simulink model "SimpleMass"  (R2018a)
settings: Solver=VariableStepAuto  StartTime=0.0  StopTime=Ttot  MaxStep=0.1  RelTol=1e-3
values from neighbouring files (symbols this model uses):
  DeadTimeValve = 0.1    [SimpleMass_Script.m]
  J = 2 * H * Sn / omegan^2    (= 4458.13208026)    [SimpleMass_Script.m]
  kgov = kgov_WHz / Sn * Fn    (= 5)    [SimpleMass_Script.m]
  Kpsec = 0    [SimpleMass_Script.m]
  omegan = 2 * pi * Fn / np    (= 314.159265359)    [SimpleMass_Script.m]
  Peini = 44e6/Sn    (= 0.5)    [SimpleMass_Script.m]
  Pestep = 4.4e6/Sn    (= 0.05)    [SimpleMass_Script.m]
  Sn = 2*44e6    (= 88000000)    [SimpleMass_Script.m]
  StepTime = 10    [SimpleMass_Script.m]
  Tgt1 = 0.1    [SimpleMass_Script.m]
  Tgt2 = 0.4    [SimpleMass_Script.m]
  Tsec = 4    [SimpleMass_Script.m]
  Tsec_on_delay = 25    [SimpleMass_Script.m]
undefined symbols (not defined in the file or in its folder): RateSec
settings Model: Creator=daniemot  LastModifiedBy=daniemot

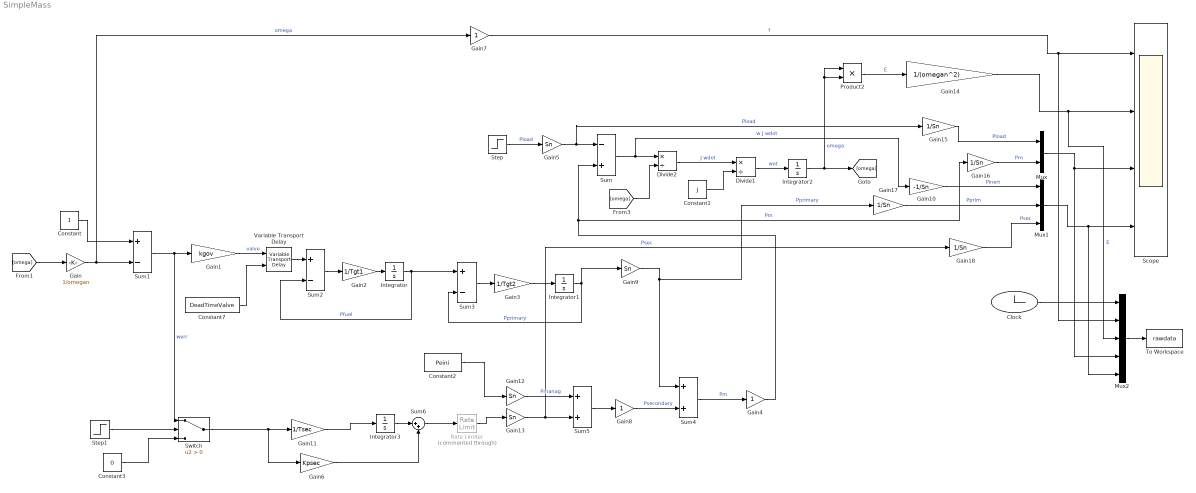
== system SimpleMass ==
  Clock : Clock
  Constant : Constant
  Constant1 : Constant  Value=J
  Constant2 : Constant  Value=Peini
  Constant3 : Constant  Value=0
  Constant7 : Constant  Value=DeadTimeValve
  Divide1 : Product  Inputs=*/
  Divide2 : Product  Inputs=*/
  Gain : Gain  Gain=1/omegan
  Gain1 : Gain  Gain=kgov
  Gain10 : Gain  Gain=-1/Sn
  Gain11 : Gain  Gain=1/Tsec
  Gain{5,9,12..13} (4 alike) : Gain  Gain=Sn
  Gain14 : Gain  Gain=1/(omegan^2)
  Gain{15..18} (4 alike) : Gain  Gain=1/Sn
  Gain2 : Gain  Gain=1/Tgt1
  Gain3 : Gain  Gain=1/Tgt2
  Gain4 : Gain
  Gain6 : Gain  Gain=Kpsec
  Gain7 : Gain
  Gain8 : Gain
  Integrator : Integrator
  Integrator1 : Integrator
  Integrator2 : Integrator  InitialCondition=omegan
  Integrator3 : Integrator
  Mux : Mux  Inputs=2
  Mux1 : Mux  Inputs=3
  Mux2 : Mux  Inputs=5
  Product2 : Product
  Rate Limiter : RateLimiter  Commented=through  RisingSlewLimit=RateSec  FallingSlewLimit=-RateSec  SampleTimeMode=inherited
  Scope : Scope  NumInputPorts=4
  Step : Step  Time=StepTime  Before=Peini  After=Peini + Pestep  SampleTime=0
  Step1 : Step  Time=Tsec_on_delay  SampleTime=0
  Sum : Sum  Inputs=-+
  Sum1 : Sum  Inputs=+-
  Sum2 : Sum  Inputs=+-
  Sum3 : Sum  Inputs=+-
  Sum4 : Sum
  Sum5 : Sum
  Sum6 : Sum  Inputs=|++
  Switch : Switch  Criteria=u2 > Threshold
  To Workspace : ToWorkspace  VariableName=rawdata  SampleTime=-1
  Variable Transport Delay : VariableTransportDelay  VariableDelayType=Variable transport delay  MaximumDelay=10  MaximumPoints=4096
  wires:
  [omega] -> Gain/1
  Gain/1 -> Sum1/2, Gain7/1  "omega"
  Constant/1 -> Sum1/1
  Sum1/1 -> Switch/1, Gain1/1  "werr"
  Gain1/1 -> Variable Transport Delay/1  "valve"
  Gain2/1 -> Integrator/1
  Sum2/1 -> Gain2/1
  Integrator1/1 -> Gain9/1, Sum3/2  "Pprimary"
  Integrator/1 -> Sum3/1, Sum2/2  "Pfuel"
  Gain3/1 -> Integrator1/1
  Sum3/1 -> Gain3/1
  Gain4/1 -> Gain16/1, Sum/2  "Pm"
  Step/1 -> Gain5/1  "Pload"
  Gain5/1 -> Gain15/1, Sum/1  "Pload"
  Divide2/1 -> Divide1/1  "J wdot"
  Constant1/1 -> Divide1/2
  Divide1/1 -> Integrator2/1  "wot"
  Integrator2/1 -> Product2/2, Product2/1, [omega]  "omega"
  Constant2/1 -> Gain12/1
  Sum4/1 -> Gain4/1  "Pm"
  [omega] -> Divide2/2
  Sum/1 -> Gain10/1, Divide2/1  "w J wdot"
  Product2/1 -> Gain14/1  "E"
  Variable Transport Delay/1 -> Sum2/1
  Constant7/1 -> Variable Transport Delay/2
  Gain7/1 -> Mux2/2, Scope/1  "f"
  Gain8/1 -> Sum4/2  "Psecondary"
  Gain9/1 -> Gain17/1, Sum4/1  "Pprimary"
  Sum5/1 -> Gain8/1
  Gain11/1 -> Integrator3/1
  Rate Limiter/1 -> Gain13/1
  Mux/1 -> Scope/3, Mux2/4
  Gain10/1 -> Mux1/1  "Pinert"
  Mux1/1 -> Mux2/5, Scope/4
  Gain12/1 -> Sum5/1  "Pmanag"
  Gain13/1 -> Gain18/1, Sum5/2  "Psec"
  Integrator3/1 -> Sum6/1
  Step1/1 -> Switch/2
  Constant3/1 -> Switch/3
  Gain14/1 -> Mux2/3, Scope/2  "E"
  Gain15/1 -> Mux/1  "Pload"
  Gain16/1 -> Mux/2  "Pm"
  Gain17/1 -> Mux1/2  "Pprim"
  Gain18/1 -> Mux1/3  "Psec"
  Mux2/1 -> To Workspace/1
  Clock/1 -> Mux2/1
  Sum6/1 -> Rate Limiter/1
  Switch/1 -> Gain11/1, Gain6/1
  Gain6/1 -> Sum6/2
